simulink model "HeadlightManagement_Project"  (R2024a)
settings: Solver=FixedStepDiscrete  StartTime=0.0  StopTime=10.0  RelTol=1e-3  EnableMultiTasking=on
undefined symbols (not defined in the file or in its folder): D1, P
libraries: autosarlibdem x1, autosarlibnvm x1
settings Model: DataDictionary=dict.sldd  Creator=Administrator  LastModifiedBy=Administrator
settings SolverCC: AlgebraicLoopSolver=TrustRegion  AutoInsertRateTranBlk=on  InsertRTBMode=Never (minimum delay)  MaxZcPerStep=1
settings OptimizationCC: DefaultParameterBehavior=Inlined  StrengthReduction=on  PassReuseOutputArgsAs=Individual arguments  ZeroExternalMemoryAtStartup=off  ZeroInternalMemoryAtStartup=off  OptimizeBlockOrder=speed  OptimizationPriority=Speed  OptimizationCustomize=off  MultiThreadedLoops=on  AutoScheduleForLoops=on  EfficientTunableParamExpr=on
settings DebuggingCC: MultiTaskDSMMsg=none  MultiTaskRateTransMsg=warning  ParameterTunabilityLossMsg=error  UnconnectedLineMsg=warning
settings SFSimCC: MATLABDynamicMemAlloc=off
settings RTWCC: Description=AUTOSAR  SystemTargetFile=autosar.tlc  GenCodeOnly=on  TemplateMakefile=ert_default_tmf  GenerateReport=on  Toolchain=MinGW64 | gmake (64-bit Windows)  IncludeHyperlinkInReport=on  LaunchReport=on  DataTypeReplacement=CDataTypesFixedWidth  CheckMdlBeforeBuild=Warning  GPUComputeCapability=3.5  DLArmComputeVersion=19.05
settings CodeAppCC: ForceParamTrailComments=on  IgnoreCustomStorageClasses=off  OperatorAnnotations=on  SimulinkDataObjDesc=on  SFDataObjDesc=on  InsertBlockDesc=on
settings STFCustomTargetCC: MultiwordLength=256  ParMdlRefBuildCompliant=on  CompOptLevelCompliant=on  IncludeMdlTerminateFcn=off  CombineOutputUpdateFcns=on  SuppressErrorStatus=on  ERTCustomFileBanners=on  SupportNonFinite=off  SupportComplex=off  SupportContinuousTime=off  SupportNonInlinedSFcns=off  RemoveResetFunc=on  MATLABClassNameForMDSCustomization=Simulink.SoftwareTarget.ERTCustomization  AutosarCompliant=on  GRTInterface=off  LookupTableObjectStructAxisOrder=2,1,3,4,...  LUTObjectStructOrderEvenSpacing=Size,Table,Breakpoints  SystemTargetFile=autosar.tlc
settings ERTTargetCC: TargetLangStandard=C99 (ISO)  ConcurrentExecutionCompliant=off  IncludeMdlTerminateFcn=off  SuppressErrorStatus=on  SupportNonFinite=off  SupportComplex=off  ModelStepFunctionPrototypeControlCompliant=off  CPPClassGenCompliant=off  AutosarCompliant=on  LookupTableObjectStructAxisOrder=2,1,3,4,...  LUTObjectStructOrderEvenSpacing=Size,Table,Breakpoints  InlinedParameterPlacement=NonHierarchical  ERTCustomFileTemplate=example_file_process.tlc  BooleanTrueId=TRUE  BooleanFalseId=FALSE

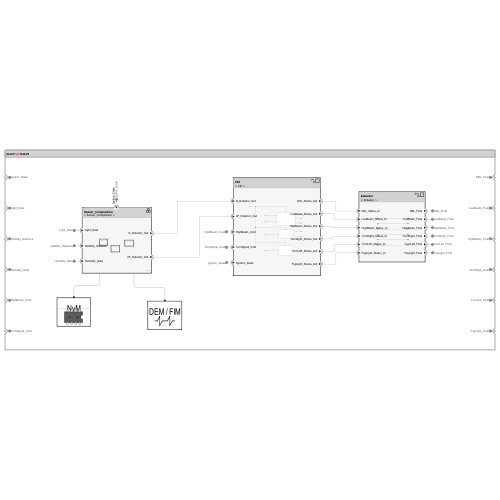
[thumbnail: Simulink's stored preview of the top-level diagram]
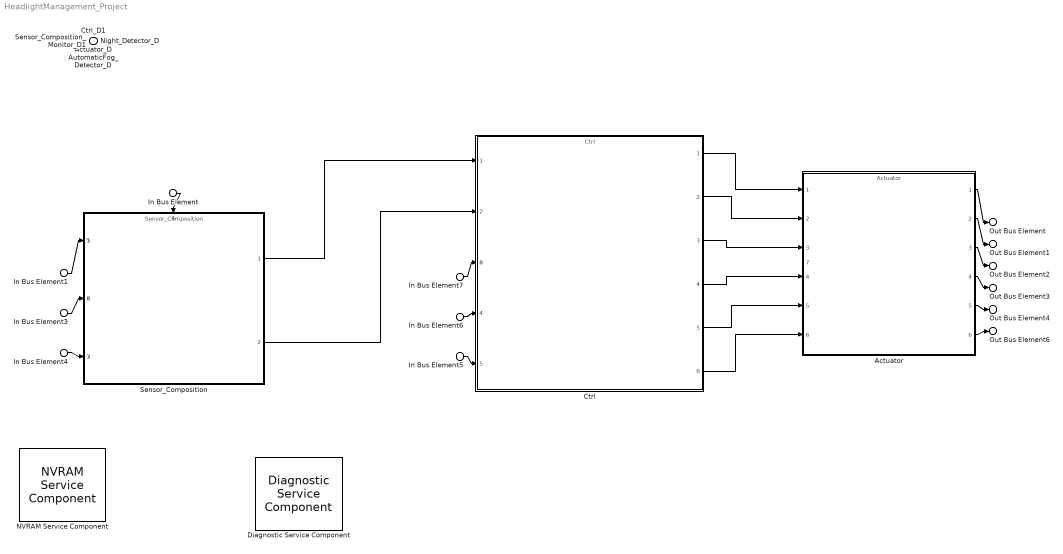
== system HeadlightManagement_Project ==
  In Bus Element : Inport  PortName=Ignition_State
  In Bus Element5 : Inport  PortName=Ignition_State
  In Bus Element1 : Inport  Port=2  PortName=Light_Data
  In Bus Element3 : Inport  Port=3  PortName=Visibility_Distance
  In Bus Element4 : Inport  Port=4  PortName=Humidity_Data
  In Bus Element7 : Inport  Port=5  PortName=HighBeam_Cmd
  In Bus Element6 : Inport  Port=6  PortName=TurnSignal_Cmd
  Actuator_D : Inport  Priority=5  Port=7  OutputFunctionCall=on
  Ctrl_D1 : Inport  Priority=4  Port=8  OutputFunctionCall=on
  AutomaticFog_Detector_D : Inport  Priority=2  Port=9  OutputFunctionCall=on
  Night_Detector_D : Inport  Priority=1  Port=10  OutputFunctionCall=on
  Sensor_Composition_Monitor_D1 : Inport  Priority=3  Port=11  OutputFunctionCall=on
  Actuator : ModelReference  ModelNameDialog=Actuator  SimulationMode=Normal  ScheduleRates=on  CachedPortDiscreteRates=[-1]  ModelEventPortInfo=P:D1[-1][0][0]  CodeInterface=Top model  ModelReferenceVersion=1.4
      settings: PortSchema="{\"entries\":[{\"content\":{\"headerSize\":38,\"margin\":15,\"minimumSpacing\":25,\"sides\":[{\"content\":{\"connectorIds\":[\"In1\",\"In2\",\"In3\",\"In4\",\"In5\",\"In6\"]},\"type\":\"ConnectorPlacement.EquallySpacedRectSide\",\"uuid\":\"5dad4047-951a-493b-8889-301a3880029f\"},{\"content\":{\"connectorIds\":[\"Out1\",\"Out2\",\"Out3\",\"Out4\",\"Out5\",\"Out6\"],\"side\":\"RIGHT\"},\"type\":\"ConnectorPlacement.EquallySpacedRectSide\",\"uuid\":\"dc227753-c29d-4407-81a4-3510fc571268\"},{\"content\":{\"side\":\"TOP\"},\"type\":\"ConnectorPlacement.EquallySpacedRectSide\",\"uuid\":\"db926774-b0ce-4057-a07c-d9fd82d8478f\"},{\"content\":{\"connectorIds\":[\"In7\"],\"side\":\"HIDDEN\"},\"type\":\"ConnectorPlacement.EquallySpacedRectSide\",\"uuid\":\"119ad781-c18d-4f41-9cbb-b55b36a667cd\"}]},\"type\":\"ConnectorPlacement.EquallySpacedConnector\",\"uuid\":\"37255525-8866-44e7-bd61-92dc9a52e660\"}],\"packageUris\":[\"http://schema.mathworks.com/mf0/Connector/R2020b\"],\"version\":\"1.0\"}"
  Ctrl : ModelReference  ModelNameDialog=Ctrl  SimulationMode=Normal  ScheduleRates=on  CachedPortDiscreteRates=[2]  ModelEventPortInfo=P:D1[2][0][0]  CodeInterface=Top model  ModelReferenceVersion=1.13
      settings: PortSchema="{\"entries\":[{\"content\":{\"headerSize\":38,\"margin\":15,\"minimumSpacing\":25,\"sides\":[{\"content\":{\"connectorIds\":[\"In1\",\"In2\",\"In3\",\"In4\",\"In5\"]},\"type\":\"ConnectorPlacement.EquallySpacedRectSide\",\"uuid\":\"5dad4047-951a-493b-8889-301a3880029f\"},{\"content\":{\"connectorIds\":[\"Out1\",\"Out2\",\"Out3\",\"Out4\",\"Out5\",\"Out6\"],\"side\":\"RIGHT\"},\"type\":\"ConnectorPlacement.EquallySpacedRectSide\",\"uuid\":\"dc227753-c29d-4407-81a4-3510fc571268\"},{\"content\":{\"side\":\"TOP\"},\"type\":\"ConnectorPlacement.EquallySpacedRectSide\",\"uuid\":\"db926774-b0ce-4057-a07c-d9fd82d8478f\"},{\"content\":{\"connectorIds\":[\"In6\"],\"side\":\"HIDDEN\"},\"type\":\"ConnectorPlacement.EquallySpacedRectSide\",\"uuid\":\"c59d87b8-e8f4-47a7-aa5c-68715c2c181d\"}]},\"type\":\"ConnectorPlacement.EquallySpacedConnector\",\"uuid\":\"37255525-8866-44e7-bd61-92dc9a52e660\"}],\"packageUris\":[\"http://schema.mathworks.com/mf0/Connector/R2020b\"],\"version\":\"1.0\"}"
  Diagnostic Service Component : autosarlibdem/Diagnostic Service Component  ClientPortNames={'AF_Detector', 'AutoFogLight_Sensor', 'N_Detector', 'Night_Sensor'}  ClientPortPortDefinedArguments={'7', '8', '5', '6'}  MaxEventId=8  MaxFID=1  DemDebounceCounterIncrementStepSize=1  DemDebounceCounterDecrementStepSize=1  DemDebounceCounterFailedThreshold=2  DemDebounceCounterPassedThreshold=-1  InhibitionMatrix=[0 0 0 0 0 0 0 0;0 0 0 0 0 0 0 0]  EnableConditionIndexes=zeros(257,'uint8')  StorageConditionIndexes=zeros(257,'uint8')
  NVRAM Service Component : autosarlibnvm/NVRAM Service Component  ClientPortNames={'Humidity_MinVal', 'Light_MinVal', 'Visibility_MinVal'}  ClientPortPortDefinedArguments={'1', '2', '3'}  MaxBlockId=10  NvInitValues={'0'}
  Sensor_Composition : ModelReference  ModelNameDialog=Sensor_Composition  SimulationMode=Normal  ScheduleRates=on  ModelReferenceVersion=1.8
      settings: PortSchema="{\"entries\":[{\"content\":{\"headerSize\":38,\"margin\":15,\"minimumSpacing\":25,\"sides\":[{\"content\":{\"connectorIds\":[\"In1\",\"In2\",\"In3\"]},\"type\":\"ConnectorPlacement.EquallySpacedRectSide\",\"uuid\":\"5dad4047-951a-493b-8889-301a3880029f\"},{\"content\":{\"connectorIds\":[\"Out1\",\"Out2\"],\"side\":\"RIGHT\"},\"type\":\"ConnectorPlacement.EquallySpacedRectSide\",\"uuid\":\"dc227753-c29d-4407-81a4-3510fc571268\"},{\"content\":{\"connectorIds\":[\"In4\"],\"side\":\"TOP\"},\"type\":\"ConnectorPlacement.EquallySpacedRectSide\",\"uuid\":\"db926774-b0ce-4057-a07c-d9fd82d8478f\"},{\"content\":{\"connectorIds\":[\"In5\",\"In6\",\"In7\"],\"side\":\"HIDDEN\"},\"type\":\"ConnectorPlacement.EquallySpacedRectSide\",\"uuid\":\"19f163bd-8bbc-4280-82cb-b83c682e2ff3\"}]},\"type\":\"ConnectorPlacement.EquallySpacedConnector\",\"uuid\":\"37255525-8866-44e7-bd61-92dc9a52e660\"}],\"packageUris\":[\"http://schema.mathworks.com/mf0/Connector/R2020b\"],\"version\":\"1.0\"}"
  Out Bus Element : Outport  PortName=DRL_Final
  Out Bus Element1 : Outport  Port=2  PortName=LowBeam_Final
  Out Bus Element2 : Outport  Port=3  PortName=HighBeam_Final
  Out Bus Element3 : Outport  Port=4  PortName=TurnRight_Final
  Out Bus Element4 : Outport  Port=5  PortName=TurnLeft_Final
  Out Bus Element6 : Outport  Port=6  PortName=FogLight_Final
  wires:
  Ctrl/6 -> Actuator/6
  In Bus Element6/1 -> Ctrl/4
  In Bus Element7/1 -> Ctrl/3
  In Bus Element5/1 -> Ctrl/5
  Ctrl/1 -> Actuator/1
  Ctrl/2 -> Actuator/2
  Ctrl/3 -> Actuator/3
  Ctrl/4 -> Actuator/4
  Ctrl/5 -> Actuator/5
  Actuator/1 -> Out Bus Element/1
  Actuator/3 -> Out Bus Element2/1
  Actuator/2 -> Out Bus Element1/1
  Actuator/6 -> Out Bus Element6/1
  Actuator/5 -> Out Bus Element4/1
  Actuator/4 -> Out Bus Element3/1
  In Bus Element4/1 -> Sensor_Composition/3
  In Bus Element/1 -> Sensor_Composition/4
  In Bus Element1/1 -> Sensor_Composition/1
  In Bus Element3/1 -> Sensor_Composition/2
  Sensor_Composition/2 -> Ctrl/2
  Sensor_Composition/1 -> Ctrl/1
